simulink model "APF_CTL_VIS_Obs_2023a"  (R2023a)
settings: Solver=ode4  StartTime=0.0  StopTime=tsim  FixedStep=baseRate  RelTol=1e-6  AbsTol=1e-6
values from neighbouring files (symbols this model uses):
  A = [0 0 0 1 0 0 ... (first row only)    [CTL_NEW.m]    (also in UKF_SPOT.m = [1 0 0 dt 0 0)
  a = 25.028    [CTL_NEW.m]
  a1 = shape(1)    [Cardioid.m]    (also in Run_Initializer.m = 0.3)
  a2 = shape(2)    [Cardioid.m]    (also in Run_Initializer.m = 0.3)
  a3 = shape(3)    [Cardioid.m]    (also in Run_Initializer.m = 0.4)
  adadelta_epsilon = 1e-5    (= 1e-05)    [Run_Initializer.m]
  adadelta_gamma = 0.37    [Run_Initializer.m]
  adagrad_epsilon = 1e-8    (= 1e-08)    [Run_Initializer.m]
  adagrad_eta = 0.18    [Run_Initializer.m]
  adam_beta_1 = 0.99    [Run_Initializer.m]
  adam_beta_2 = 0.999    [Run_Initializer.m]
  adam_epsilon = 1e-2    (= 0.01)    [Run_Initializer.m]
  adam_eta = 0.0163    [Run_Initializer.m]
  adamax_beta_1 = 0.5    [Run_Initializer.m]
  adamax_beta_2 = 0.999    [Run_Initializer.m]
  adamax_eta = 0.014    [Run_Initializer.m]
  alpha_Black = 0.9    [UKF_SPOT.m]
  alpha_Blue = 0.9    [UKF_SPOT.m]
  Att_Mode = 0    [Run_Initializer.m]
  b1 = shape(4)    [Cardioid.m]    (also in Run_Initializer.m = 0.175)
  b2 = shape(5)    [Cardioid.m]    (also in Run_Initializer.m = 0.175)
  beta_Black = 2    [UKF_SPOT.m]
  beta_Blue = 20    [UKF_SPOT.m]
  Binv = inv(B)    [Run_Initializer.m]
  BLACK_end = [2, 1.4, deg2rad(368)]    [Run_Initializer.m]
  BLACK_ini = [2, 1.4, deg2rad(188), 0, 0, deg2rad(1.5)]    [Run_Initializer.m]
  BLUE_end = [1.3, 1.25, deg2rad(90)]    [Run_Initializer.m]
  BLUE_ini = [1.3, 1.25, deg2rad(270), 0, 0, deg2rad(-1.5)]    [Run_Initializer.m]
  drop_states_BLACK = BLACK_ini(1:3)    [Run_Initializer.m]
  drop_states_BLUE = BLUE_ini(1:3)    [Run_Initializer.m]
  drop_states_RED = RED_ini(1:3)    [Run_Initializer.m]
  dt = 0.01    [UKF_SPOT.m]
  end_time_black = 300    [Run_Initializer.m]
  end_time_blue = 300    [Run_Initializer.m]
  F_max = 0.22    [CTL_NEW.m]
  Gamma1_el = 0.12    [Run_Initializer.m]
  Gamma1_sh = 0.005    [Run_Initializer.m]
  Gamma1_wr = 0.025    [Run_Initializer.m]
  Gamma2_el = 5    [Run_Initializer.m]
  Gamma2_sh = 5    [Run_Initializer.m]
  Gamma2_wr = 5    [Run_Initializer.m]
  Gamma3_el = 10    [Run_Initializer.m]
  Gamma3_sh = 40    [Run_Initializer.m]
  Gamma3_wr = 40    [Run_Initializer.m]
  Gamma4_el = 0.039    [Run_Initializer.m]
  Gamma4_sh = 0.015    [Run_Initializer.m]
  Gamma4_wr = 0.029    [Run_Initializer.m]
  Gamma5_el = 800    [Run_Initializer.m]
  Gamma5_sh = 800    [Run_Initializer.m]
  Gamma5_wr = 800    [Run_Initializer.m]
  Gamma6_el = 0.000001    (= 1e-06)    [Run_Initializer.m]
  Gamma6_sh = 0.005    [Run_Initializer.m]
  Gamma6_wr = 0.02    [Run_Initializer.m]
  H = [1 0 0 0 0 0 ... (first row only)    [UKF_SPOT.m]
  home_states_BLACK = BLACK_ini(1:3)    [Run_Initializer.m]
  home_states_BLUE = BLUE_ini(1:3)    [Run_Initializer.m]
  home_states_RED = RED_ini(1:3)    [Run_Initializer.m]
  Hz = 0.01    [CTL_NEW.m]
  init_states_BLACK = BLACK_ini(1:3)    [Run_Initializer.m]
  init_states_BLUE = BLUE_ini(1:3)    [Run_Initializer.m]
  init_states_RED = RED_ini(1:3)    [Run_Initializer.m]
  J = IRED    [CTL_NEW.m]    (also in UKF_SPOT.m = 0.20184)
  k = lqr(A,B1,Q,R)    [CTL_NEW.m]
  k_1_0 = k(1,1)    [CTL_NEW.m]
  k_1_t_0 = k(3,3)    [CTL_NEW.m]
  k_2_0 = k(1,4)    [CTL_NEW.m]
  k_2_t_0 = k(3,6)    [CTL_NEW.m]
  K_a = diag([2 2 3.5])    [Run_Initializer.m]
  ka = 1    [Run_Initializer.m]
  Kd_elarm = 0.8    [Run_Initializer.m]
  Kd_sharm = 1.0    (= 1)    [Run_Initializer.m]
  Kd_t = 9.5    [CTL_NEW.m]    (also in Run_Initializer.m)
  Kd_wrarm = 0.6    [Run_Initializer.m]
  Kd_x = 28    [CTL_NEW.m]    (also in Run_Initializer.m)
  Kd_y = Kd_x    (= 28)    [CTL_NEW.m]    (also in Run_Initializer.m)
  Kp_elarm = 1.2    [Run_Initializer.m]
  Kp_sharm = 1.5    [Run_Initializer.m]
  Kp_t = 1    [CTL_NEW.m]    (also in Run_Initializer.m)
  Kp_wrarm = 2    [Run_Initializer.m]
  Kp_x = 3.5    [CTL_NEW.m]    (also in Run_Initializer.m)
  Kp_y = Kp_x    (= 3.5)    [CTL_NEW.m]    (also in Run_Initializer.m)
  kr = 2    [Run_Initializer.m]
  lambda1 = 0.4    [CTL_NEW.m]
  lambda12 = 0.4    [CTL_NEW.m]
  lambda12_t = 0.05    [CTL_NEW.m]
  lambda1_t = 0.05    [CTL_NEW.m]
  lambda2 = 0.4    [CTL_NEW.m]
  lambda2_t = 0.05    [CTL_NEW.m]
  lamda_Black = (alpha_Black^2)*(N + kappa_Black) - N    (= 15.06)    [UKF_SPOT.m]
  lamda_Blue = (alpha_Blue^2)*(N + kappa_Blue) - N    (= 6.96)    [UKF_SPOT.m]
  m = mRED    [CTL_NEW.m]    (also in UKF_SPOT.m = 11.21)
  method = 1    [UKF_SPOT.m]
  Method = 8    [Run_Initializer.m]
  momentum_eta = 0.7    [Run_Initializer.m]
  momentum_gamma = 0.7    [Run_Initializer.m]
  nesterov_eta = 0.6    [Run_Initializer.m]
  nesterov_gamma = 0.3    [Run_Initializer.m]
  Nmat = diag([1 1 1])    [Run_Initializer.m]
  p = 0.4    [CTL_NEW.m]
  P_b = diag([45 45 0])    [Run_Initializer.m]
  P_IC_Black = 0.2*eye(6)    [UKF_SPOT.m]
  P_IC_Blue = 0.2*eye(6)    [UKF_SPOT.m]
  p_t = 0.05    [CTL_NEW.m]
  psi = 1    [Run_Initializer.m]
  PWMFreq = 5    [Run_Initializer.m]
  Q = [w 0 0 0 0 0 ... (first row only)    [CTL_NEW.m]
  Q_a = diag([5, 5, 0])    [Run_Initializer.m]
  Q_b = diag([0.0125, 0.0125, 0.05])    [Run_Initializer.m]
  Q_Black = [0.0000005 0 0 0 0 0 ... (first row only)    [UKF_SPOT.m]
  Q_Blue = [0.000075 0 0 0 0 0 ... (first row only)    [UKF_SPOT.m]
  R = [r 0 0 ... (first row only)    [CTL_NEW.m]
  R_Black = [variance 0 0 ... (first row only)    [UKF_SPOT.m]
  R_Blue = [variance 0 0 ... (first row only)    [UKF_SPOT.m]
  r_hold = 0.427    [Run_Initializer.m]
  r_off = 0.165    [Run_Initializer.m]
  RED_ini = [2.7, 0.4, deg2rad(135+360), 0, 0, 0]    [Run_Initializer.m]
  Red_Rate = 0.025    [CTL_NEW.m]
  RMSprop_epsilon = 1e-8    (= 1e-08)    [Run_Initializer.m]
  RMSprop_eta = 0.025    [Run_Initializer.m]
  RMSprop_gamma = 0.9    [Run_Initializer.m]
  ... (+11 more)
undefined symbols (not defined in the file or in its folder): alpha, alpha_m, alphap, alphat, Am, b, b0, b3, baseRate, beta, Bm, c, Cm, d, DiscIntNeverNeededParam, Dm, drop_states_ARM, epsilon, F_Black_X_nominal, F_Black_Y_nominal, F_Blue_X_nominal, F_Blue_Y_nominal, F_red_X_nominal, F_red_Y_nominal, F_thrusters_BLACK, F_thrusters_BLUE, F_thrusters_RED, IBLACK, IBLUE, IDIST, IEE, IPROX, IRED, K, k1, k1t, k2, k2t, K_t, Kd_tb, Kd_tblue, Kd_tr, Kd_xb, Kd_xblue, Kd_xr, Kd_yb, Kd_yblue, Kd_yr, Kp_tb, Kp_tblue, Kp_tr, Kp_xb, Kp_xblue, Kp_xr, Kp_yb, Kp_yblue, Kp_yr, lamda ... (+34)
libraries: nvidiaSharedBlocks x10, MainLibrary x4, dspsigops x4, simulink x2, etargetslib x1
(part 11 of 15)

== system APF_CTL_VIS_Obs_2023a/Phase #3: Experiment/Change RED Behavior/Sub-Phase #3 /Custom Discrete PD (Attitude)/x_dot -> x2/Hold this value ==
  In1 : Inport
  Action Port : ActionPort  ActionPortLabel=if(u1 ~= 0)
  Out1 : Outport  VectorParamsAs1DForOutWhenUnconnected=off
  wires:
  In1/1 -> Out1/1

== system APF_CTL_VIS_Obs_2023a/Phase #3: Experiment/Change RED Behavior/Sub-Phase #3 /Custom Discrete PD (X-Position)/x_dot -> x2/Hold this value ==
  In1 : Inport
  Action Port : ActionPort  ActionPortLabel=if(u1 ~= 0)
  Out1 : Outport  VectorParamsAs1DForOutWhenUnconnected=off
  wires:
  In1/1 -> Out1/1

== system APF_CTL_VIS_Obs_2023a/Phase #3: Experiment/Change RED Behavior/Sub-Phase #3 /Custom Discrete PD (Y-Position)/x_dot -> x2/Hold this value ==
  In1 : Inport
  Action Port : ActionPort  ActionPortLabel=if(u1 ~= 0)
  Out1 : Outport  VectorParamsAs1DForOutWhenUnconnected=off
  wires:
  In1/1 -> Out1/1

== system APF_CTL_VIS_Obs_2023a/Phase #3: Experiment/Change RED Behavior/Sub-Phase #3 /RED+ARM/Simulated Position Controller/Custom Discrete PD (Elbow) ==
  ey : Inport
  Sum3 : Sum
  kd_elarm : Gain  Gain=Kd_elarm
  kp_elarm : Gain  Gain=Kp_elarm
  "x_dot -> x2" : Subsystem
  Fy : Outport  VectorParamsAs1DForOutWhenUnconnected=off
  wires:
  kd_elarm/1 -> Sum3/1
  Sum3/1 -> Fy/1
  kp_elarm/1 -> Sum3/2
  "x_dot -> x2"/1(dy(t)/dt) -> kd_elarm/1
  ey/1 -> "x_dot -> x2"/1(y(t)), kp_elarm/1

== system APF_CTL_VIS_Obs_2023a/Phase #3: Experiment/Change RED Behavior/Sub-Phase #3 /RED+ARM/Simulated Position Controller/Custom Discrete PD (Shoulder) ==
  ex : Inport
  Sum3 : Sum
  kd_sharm : Gain  Gain=Kd_sharm
  kp_sharm : Gain  Gain=Kp_sharm
  "x_dot -> x2" : Subsystem
  Fx : Outport  VectorParamsAs1DForOutWhenUnconnected=off
  wires:
  kd_sharm/1 -> Sum3/1
  ex/1 -> "x_dot -> x2"/1(y(t)), kp_sharm/1
  kp_sharm/1 -> Sum3/2
  "x_dot -> x2"/1(dy(t)/dt) -> kd_sharm/1
  Sum3/1 -> Fx/1

== system APF_CTL_VIS_Obs_2023a/Phase #3: Experiment/Change RED Behavior/Sub-Phase #3 /RED+ARM/Simulated Position Controller/Custom Discrete PD (Wrist) ==
  ey : Inport
  Sum3 : Sum
  kd_wrarm : Gain  Gain=Kd_wrarm
  kp_wrarm : Gain  Gain=Kp_wrarm
  "x_dot -> x2" : Subsystem
  Fy : Outport  VectorParamsAs1DForOutWhenUnconnected=off
  wires:
  kd_wrarm/1 -> Sum3/1
  Sum3/1 -> Fy/1
  kp_wrarm/1 -> Sum3/2
  "x_dot -> x2"/1(dy(t)/dt) -> kd_wrarm/1
  ey/1 -> "x_dot -> x2"/1(y(t)), kp_wrarm/1

== system APF_CTL_VIS_Obs_2023a/Phase #3: Experiment/Change RED Behavior/Sub-Phase #4/CTL/If Action Subsystem/CSMC3 ==
  note: epsilon = 2*u_max
  note: k = mass, but i may make it variable for performance
  note: alpha = variable
  e_x : Inport
  e_y : Inport  Port=2
  e_t : Inport  Port=3
  Derivative : Derivative
  Derivative1 : Derivative
  Derivative2 : Derivative
  MATLAB Function : MATLAB Function  TreatAsAtomicUnit=on
  MATLAB Function1 : MATLAB Function  TreatAsAtomicUnit=on
  MATLAB Function2 : MATLAB Function  TreatAsAtomicUnit=on
  MATLAB Function3 : MATLAB Function  TreatAsAtomicUnit=on
  MATLAB Function4 : MATLAB Function  TreatAsAtomicUnit=on
  MATLAB Function5 : MATLAB Function  TreatAsAtomicUnit=on
  MATLAB Function6 : MATLAB Function  TreatAsAtomicUnit=on
  MATLAB Function7 : MATLAB Function  TreatAsAtomicUnit=on
  MATLAB Function8 : MATLAB Function  TreatAsAtomicUnit=on
  Saturation{,1..5} (6 alike) : Saturate  UpperLimit=epsilon  LowerLimit=-epsilon
  Sum : Sum  Inputs=++|
  Sum1 : Sum  Inputs=++|
  Sum2 : Sum  Inputs=++|
  F_x : Outport
  F_y : Outport  Port=2
  tau : Outport  Port=3
  wires:
  Sum2/1 -> tau/1
  MATLAB Function6/1(u) -> Saturation5/1
  MATLAB Function8/1(phi) -> MATLAB Function6/1(phi)
  Derivative2/1 -> MATLAB Function8/2(q2), MATLAB Function7/1(q2)
  Saturation5/1 -> Sum2/1
  Saturation4/1 -> Sum2/2
  MATLAB Function7/1(u) -> Saturation4/1
  e_t/1 -> Derivative2/1, MATLAB Function8/1(q1)
  Sum1/1 -> F_y/1
  MATLAB Function3/1(u) -> Saturation3/1
  MATLAB Function4/1(u) -> Saturation2/1
  Derivative1/1 -> MATLAB Function4/1(q2), MATLAB Function5/2(q2)
  e_y/1 -> MATLAB Function5/1(q1), Derivative1/1
  Saturation3/1 -> Sum1/1
  MATLAB Function5/1(phi) -> MATLAB Function3/1(phi)
  Saturation2/1 -> Sum1/2
  Saturation1/1 -> Sum/1
  Saturation/1 -> Sum/2
  MATLAB Function2/1(phi) -> MATLAB Function/1(phi)
  MATLAB Function1/1(u) -> Saturation/1
  MATLAB Function/1(u) -> Saturation1/1
  Sum/1 -> F_x/1
  Derivative/1 -> MATLAB Function1/1(q2), MATLAB Function2/2(q2)
  e_x/1 -> Derivative/1, MATLAB Function2/1(q1)

== system APF_CTL_VIS_Obs_2023a/Phase #3: Experiment/Change RED Behavior/Sub-Phase #4/CTL/If Action Subsystem/DAC Controller1 ==
  e_x : Inport
  In2 : Inport  Port=2
  e_t : Inport  Port=3
  Add2 : Sum
  Derivative1 : Derivative
  Derivative2 : Derivative
  Derivative3 : Derivative
  Discrete-Time Integrator : DiscreteIntegrator  InitialCondition=k_2_t_0  SampleTime=-1  ICPrevOutput=DiscIntNeverNeededParam  ICPrevScaledInput=DiscIntNeverNeededParam
  Discrete-Time Integrator1 : DiscreteIntegrator  InitialCondition=k_1_t_0  SampleTime=-1  ICPrevOutput=DiscIntNeverNeededParam  ICPrevScaledInput=DiscIntNeverNeededParam
  Discrete-Time Integrator2 : DiscreteIntegrator  InitialCondition=k_2_0  SampleTime=-1  ICPrevOutput=DiscIntNeverNeededParam  ICPrevScaledInput=DiscIntNeverNeededParam
  Discrete-Time Integrator3 : DiscreteIntegrator  InitialCondition=k_1_0  SampleTime=-1  ICPrevOutput=DiscIntNeverNeededParam  ICPrevScaledInput=DiscIntNeverNeededParam
  Discrete-Time Integrator4 : DiscreteIntegrator  InitialCondition=k_2_0  SampleTime=-1  ICPrevOutput=DiscIntNeverNeededParam  ICPrevScaledInput=DiscIntNeverNeededParam
  Discrete-Time Integrator5 : DiscreteIntegrator  InitialCondition=k_1_0  SampleTime=-1  ICPrevOutput=DiscIntNeverNeededParam  ICPrevScaledInput=DiscIntNeverNeededParam
  Fx Gain Derivatives : MATLAB Function  TreatAsAtomicUnit=on
  Fy Gain Derivatives : MATLAB Function  TreatAsAtomicUnit=on
  Product4 : Product
  Product5 : Product
  Pseudo Derivative2 : TransferFcn  Commented=on  Numerator=[a 0]  Denominator=[1 a]
  Torque Gain Derivatives : MATLAB Function  TreatAsAtomicUnit=on
  k_1*q_1_x : Product
  k_1*q_1_y : Product
  k_2*q2_x : Product
  k_2*q2_y : Product
  u_x : Sum
  u_y : Sum
  Out1 : Outport
  Out2 : Outport  Port=2
  Out3 : Outport  Port=3
  wires:
  u_y/1 -> Out2/1
  Discrete-Time Integrator3/1 -> k_1*q_1_y/1
  Derivative1/1 -> k_2*q2_y/1, Fy Gain Derivatives/1(e_ydot)
  In2/1 -> Derivative1/1, Fy Gain Derivatives/2(e_y), k_1*q_1_y/2
  k_2*q2_y/1 -> u_y/1
  Fy Gain Derivatives/2(k1_dot) -> Discrete-Time Integrator3/1
  Discrete-Time Integrator2/1 -> k_2*q2_y/2
  k_1*q_1_y/1 -> u_y/2
  Fy Gain Derivatives/1(k2_dot) -> Discrete-Time Integrator2/1
  Discrete-Time Integrator1/1 -> Product5/2
  Torque Gain Derivatives/1(k1_dot) -> Discrete-Time Integrator1/1
  Derivative3/1 -> Product4/2, Torque Gain Derivatives/2(e_tdot)
  Discrete-Time Integrator/1 -> Product4/1
  Product5/1 -> Add2/1
  Product4/1 -> Add2/2
  Torque Gain Derivatives/2(k2_dot) -> Discrete-Time Integrator/1
  Add2/1 -> Out3/1
  e_x/1 -> Derivative2/1, k_1*q_1_x/2, Fx Gain Derivatives/2(e_x)
  Discrete-Time Integrator4/1 -> k_2*q2_x/2
  Discrete-Time Integrator5/1 -> k_1*q_1_x/1
  Fx Gain Derivatives/2(k1_dot) -> Discrete-Time Integrator5/1
  Fx Gain Derivatives/1(k2_dot) -> Discrete-Time Integrator4/1
  Derivative2/1 -> k_2*q2_x/1, Fx Gain Derivatives/1(e_xdot)
  k_1*q_1_x/1 -> u_x/2
  u_x/1 -> Out1/1
  k_2*q2_x/1 -> u_x/1
  e_t/1 -> Product5/1, Derivative3/1, Torque Gain Derivatives/1(e_t)

== system APF_CTL_VIS_Obs_2023a/Phase #3: Experiment/Change RED Behavior/Sub-Phase #4/CTL/If Action Subsystem/DAC Controller2 ==
  e_x : Inport
  In2 : Inport  Port=2
  e_t : Inport  Port=3
  Add2 : Sum
  Derivative1 : Derivative
  Derivative2 : Derivative
  Derivative3 : Derivative
  Discrete-Time Integrator : DiscreteIntegrator  InitialCondition=k_2_t_0  SampleTime=-1  ICPrevOutput=DiscIntNeverNeededParam  ICPrevScaledInput=DiscIntNeverNeededParam
  Discrete-Time Integrator1 : DiscreteIntegrator  InitialCondition=k_1_t_0  SampleTime=-1  ICPrevOutput=DiscIntNeverNeededParam  ICPrevScaledInput=DiscIntNeverNeededParam
  Discrete-Time Integrator2 : DiscreteIntegrator  InitialCondition=k_2_0  SampleTime=-1  ICPrevOutput=DiscIntNeverNeededParam  ICPrevScaledInput=DiscIntNeverNeededParam
  Discrete-Time Integrator3 : DiscreteIntegrator  InitialCondition=k_1_0  SampleTime=-1  ICPrevOutput=DiscIntNeverNeededParam  ICPrevScaledInput=DiscIntNeverNeededParam
  Discrete-Time Integrator4 : DiscreteIntegrator  InitialCondition=k_2_0  SampleTime=-1  ICPrevOutput=DiscIntNeverNeededParam  ICPrevScaledInput=DiscIntNeverNeededParam
  Discrete-Time Integrator5 : DiscreteIntegrator  InitialCondition=k_1_0  SampleTime=-1  ICPrevOutput=DiscIntNeverNeededParam  ICPrevScaledInput=DiscIntNeverNeededParam
  Fx Gain Derivatives : MATLAB Function  TreatAsAtomicUnit=on
  Fy Gain Derivatives : MATLAB Function  TreatAsAtomicUnit=on
  Product4 : Product
  Product5 : Product
  Pseudo Derivative2 : TransferFcn  Commented=on  Numerator=[a 0]  Denominator=[1 a]
  Torque Gain Derivatives : MATLAB Function  TreatAsAtomicUnit=on
  k_1*q_1_x : Product
  k_1*q_1_y : Product
  k_2*q2_x : Product
  k_2*q2_y : Product
  u_x : Sum
  u_y : Sum
  Out1 : Outport
  Out2 : Outport  Port=2
  Out3 : Outport  Port=3
  wires:
  e_t/1 -> Torque Gain Derivatives/1(e_t), Derivative3/1, Product5/1
  k_2*q2_x/1 -> u_x/1
  u_x/1 -> Out1/1
  k_1*q_1_x/1 -> u_x/2
  Derivative2/1 -> Fx Gain Derivatives/1(e_xdot), k_2*q2_x/1
  Fx Gain Derivatives/1(k2_dot) -> Discrete-Time Integrator4/1
  Fx Gain Derivatives/2(k1_dot) -> Discrete-Time Integrator5/1
  Discrete-Time Integrator5/1 -> k_1*q_1_x/1
  Discrete-Time Integrator4/1 -> k_2*q2_x/2
  e_x/1 -> Fx Gain Derivatives/2(e_x), k_1*q_1_x/2, Derivative2/1
  Add2/1 -> Out3/1
  Torque Gain Derivatives/2(k2_dot) -> Discrete-Time Integrator/1
  Product4/1 -> Add2/2
  Product5/1 -> Add2/1
  Discrete-Time Integrator/1 -> Product4/1
  Derivative3/1 -> Torque Gain Derivatives/2(e_tdot), Product4/2
  Torque Gain Derivatives/1(k1_dot) -> Discrete-Time Integrator1/1
  Discrete-Time Integrator1/1 -> Product5/2
  Fy Gain Derivatives/1(k2_dot) -> Discrete-Time Integrator2/1
  k_1*q_1_y/1 -> u_y/2
  Discrete-Time Integrator2/1 -> k_2*q2_y/2
  Fy Gain Derivatives/2(k1_dot) -> Discrete-Time Integrator3/1
  k_2*q2_y/1 -> u_y/1
  In2/1 -> k_1*q_1_y/2, Fy Gain Derivatives/2(e_y), Derivative1/1
  Derivative1/1 -> Fy Gain Derivatives/1(e_ydot), k_2*q2_y/1
  Discrete-Time Integrator3/1 -> k_1*q_1_y/1
  u_y/1 -> Out2/1

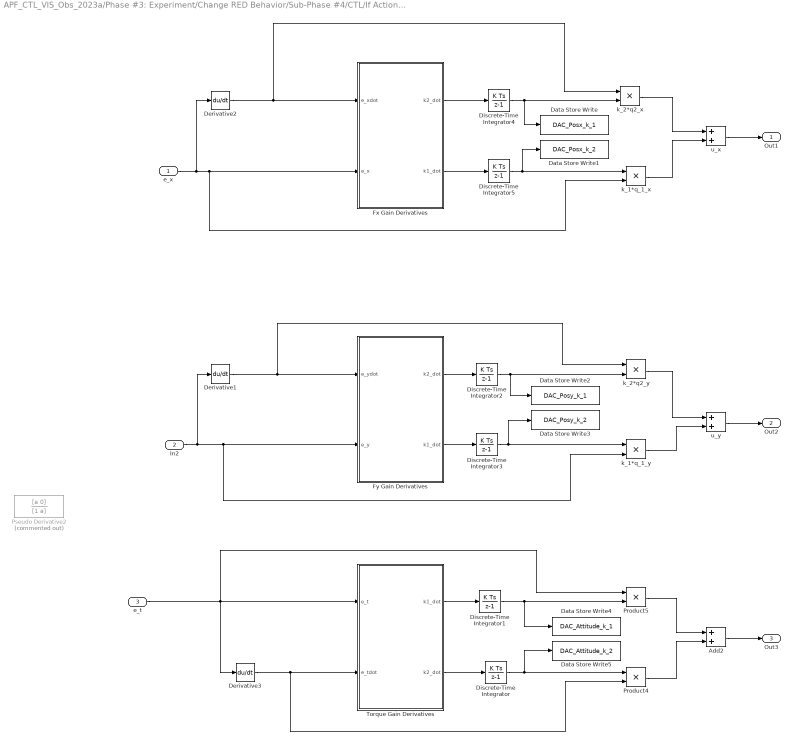
== system APF_CTL_VIS_Obs_2023a/Phase #3: Experiment/Change RED Behavior/Sub-Phase #4/CTL/If Action Subsystem/DAC Controller3 ==
  e_x : Inport
  In2 : Inport  Port=2
  e_t : Inport  Port=3
  Add2 : Sum
  Data Store Write : DataStoreWrite  DataStoreName=DAC_Posx_k_1  IndexOptions=Index vector (dialog)  Indices=1  OutputSizes=1
  Data Store Write1 : DataStoreWrite  DataStoreName=DAC_Posx_k_2  IndexOptions=Index vector (dialog)  Indices=1  OutputSizes=1
  Data Store Write2 : DataStoreWrite  DataStoreName=DAC_Posy_k_1  IndexOptions=Index vector (dialog)  Indices=1  OutputSizes=1
  Data Store Write3 : DataStoreWrite  DataStoreName=DAC_Posy_k_2  IndexOptions=Index vector (dialog)  Indices=1  OutputSizes=1
  Data Store Write4 : DataStoreWrite  DataStoreName=DAC_Attitude_k_1  IndexOptions=Index vector (dialog)  Indices=1  OutputSizes=1
  Data Store Write5 : DataStoreWrite  DataStoreName=DAC_Attitude_k_2  IndexOptions=Index vector (dialog)  Indices=1  OutputSizes=1
  Derivative1 : Derivative
  Derivative2 : Derivative
  Derivative3 : Derivative
  Discrete-Time Integrator : DiscreteIntegrator  InitialCondition=k_2_t_0  SampleTime=-1  ICPrevOutput=DiscIntNeverNeededParam  ICPrevScaledInput=DiscIntNeverNeededParam
  Discrete-Time Integrator1 : DiscreteIntegrator  InitialCondition=k_1_t_0  SampleTime=-1  ICPrevOutput=DiscIntNeverNeededParam  ICPrevScaledInput=DiscIntNeverNeededParam
  Discrete-Time Integrator2 : DiscreteIntegrator  InitialCondition=k_2_0  SampleTime=-1  ICPrevOutput=DiscIntNeverNeededParam  ICPrevScaledInput=DiscIntNeverNeededParam
  Discrete-Time Integrator3 : DiscreteIntegrator  InitialCondition=k_1_0  SampleTime=-1  ICPrevOutput=DiscIntNeverNeededParam  ICPrevScaledInput=DiscIntNeverNeededParam
  Discrete-Time Integrator4 : DiscreteIntegrator  InitialCondition=k_2_0  SampleTime=-1  ICPrevOutput=DiscIntNeverNeededParam  ICPrevScaledInput=DiscIntNeverNeededParam
  Discrete-Time Integrator5 : DiscreteIntegrator  InitialCondition=k_1_0  SampleTime=-1  ICPrevOutput=DiscIntNeverNeededParam  ICPrevScaledInput=DiscIntNeverNeededParam
  Fx Gain Derivatives : MATLAB Function  TreatAsAtomicUnit=on
  Fy Gain Derivatives : MATLAB Function  TreatAsAtomicUnit=on
  Product4 : Product
  Product5 : Product
  Pseudo Derivative2 : TransferFcn  Commented=on  Numerator=[a 0]  Denominator=[1 a]
  Torque Gain Derivatives : MATLAB Function  TreatAsAtomicUnit=on
  k_1*q_1_x : Product
  k_1*q_1_y : Product
  k_2*q2_x : Product
  k_2*q2_y : Product
  u_x : Sum
  u_y : Sum
  Out1 : Outport
  Out2 : Outport  Port=2
  Out3 : Outport  Port=3
  wires:
  u_y/1 -> Out2/1
  Discrete-Time Integrator3/1 -> Data Store Write3/1, k_1*q_1_y/1
  Derivative1/1 -> k_2*q2_y/1, Fy Gain Derivatives/1(e_ydot)
  In2/1 -> Derivative1/1, Fy Gain Derivatives/2(e_y), k_1*q_1_y/2
  k_2*q2_y/1 -> u_y/1
  Fy Gain Derivatives/2(k1_dot) -> Discrete-Time Integrator3/1
  Discrete-Time Integrator2/1 -> Data Store Write2/1, k_2*q2_y/2
  k_1*q_1_y/1 -> u_y/2
  Fy Gain Derivatives/1(k2_dot) -> Discrete-Time Integrator2/1
  Discrete-Time Integrator1/1 -> Data Store Write4/1, Product5/2
  Torque Gain Derivatives/1(k1_dot) -> Discrete-Time Integrator1/1
  Derivative3/1 -> Product4/2, Torque Gain Derivatives/2(e_tdot)
  Discrete-Time Integrator/1 -> Data Store Write5/1, Product4/1
  Product5/1 -> Add2/1
  Product4/1 -> Add2/2
  Torque Gain Derivatives/2(k2_dot) -> Discrete-Time Integrator/1
  Add2/1 -> Out3/1
  e_x/1 -> Derivative2/1, k_1*q_1_x/2, Fx Gain Derivatives/2(e_x)
  Discrete-Time Integrator4/1 -> Data Store Write/1, k_2*q2_x/2
  Discrete-Time Integrator5/1 -> Data Store Write1/1, k_1*q_1_x/1
  Fx Gain Derivatives/2(k1_dot) -> Discrete-Time Integrator5/1
  Fx Gain Derivatives/1(k2_dot) -> Discrete-Time Integrator4/1
  Derivative2/1 -> k_2*q2_x/1, Fx Gain Derivatives/1(e_xdot)
  k_1*q_1_x/1 -> u_x/2
  u_x/1 -> Out1/1
  k_2*q2_x/1 -> u_x/1
  e_t/1 -> Product5/1, Derivative3/1, Torque Gain Derivatives/1(e_t)

== system APF_CTL_VIS_Obs_2023a/Phase #3: Experiment/Change RED Behavior/Sub-Phase #4/CTL/If Action Subsystem/H_inf ==
  e_x : Inport
  e_y : Inport  Port=2
  e_t : Inport  Port=3
  H Infinity (Attitude) : Subsystem
  H Infinity (X-Position) : Subsystem
  H Infinity (Y-Position) : Subsystem
  F_x : Outport
  F_y : Outport  Port=2
  tau : Outport  Port=3
  wires:
  e_x/1 -> H Infinity (X-Position)/1(ex)
  e_y/1 -> H Infinity (Y-Position)/1(ey)
  e_t/1 -> H Infinity (Attitude)/1(ez)
  H Infinity (Attitude)/1(Tz) -> tau/1
  H Infinity (Y-Position)/1(Fy) -> F_y/1
  H Infinity (X-Position)/1(Fx) -> F_x/1

== system APF_CTL_VIS_Obs_2023a/Phase #3: Experiment/Change RED Behavior/Sub-Phase #4/CTL/If Action Subsystem/Homo ==
  e_x : Inport
  e_y : Inport  Port=2
  e_t : Inport  Port=3
  Derivative : Derivative
  Derivative1 : Derivative
  Derivative2 : Derivative
  MATLAB Function : MATLAB Function  TreatAsAtomicUnit=on
  MATLAB Function1 : MATLAB Function  TreatAsAtomicUnit=on
  MATLAB Function2 : MATLAB Function  TreatAsAtomicUnit=on
  MATLAB Function3 : MATLAB Function  TreatAsAtomicUnit=on
  MATLAB Function4 : MATLAB Function  TreatAsAtomicUnit=on
  MATLAB Function5 : MATLAB Function  TreatAsAtomicUnit=on
  Sum : Sum  Inputs=++|
  Sum1 : Sum  Inputs=++|
  Sum2 : Sum  Inputs=++|
  F_x : Outport
  F_y : Outport  Port=2
  tau : Outport  Port=3
  wires:
  e_x/1 -> Derivative2/1, MATLAB Function/1(q1)
  Derivative2/1 -> MATLAB Function1/1(q2)
  Sum/1 -> F_x/1
  MATLAB Function/1(u) -> Sum/1
  MATLAB Function1/1(u) -> Sum/2
  Derivative1/1 -> MATLAB Function3/1(q2)
  Sum1/1 -> F_y/1
  MATLAB Function3/1(u) -> Sum1/2
  e_y/1 -> Derivative1/1, MATLAB Function2/1(q1)
  MATLAB Function2/1(u) -> Sum1/1
  e_t/1 -> Derivative/1, MATLAB Function4/1(q1)
  Derivative/1 -> MATLAB Function5/1(q2)
  MATLAB Function5/1(u) -> Sum2/2
  MATLAB Function4/1(u) -> Sum2/1
  Sum2/1 -> tau/1

== system APF_CTL_VIS_Obs_2023a/Phase #3: Experiment/Change RED Behavior/Sub-Phase #4/CTL/If Action Subsystem/LQR ==
  e_x : Inport
  e_y : Inport  Port=2
  e_t : Inport  Port=3
  Constant : Constant  Value=k
  Demux : Demux  Outputs=3
  Derivative : Derivative
  Derivative1 : Derivative
  Derivative2 : Derivative
  MATLAB Function : MATLAB Function  TreatAsAtomicUnit=on
  F_x : Outport
  F_y : Outport  Port=2
  tau : Outport  Port=3
  wires:
  Constant/1 -> MATLAB Function/1(k)
  MATLAB Function/1(u) -> Demux/1
  Demux/2 -> F_y/1
  Demux/1 -> F_x/1
  Demux/3 -> tau/1
  e_t/1 -> MATLAB Function/6(q1_t), Derivative/1
  e_y/1 -> Derivative1/1, MATLAB Function/4(q1_y)
  e_x/1 -> Derivative2/1, MATLAB Function/2(q1_x)
  Derivative/1 -> MATLAB Function/7(q2_t)
  Derivative1/1 -> MATLAB Function/5(q2_y)
  Derivative2/1 -> MATLAB Function/3(q2_x)

== system APF_CTL_VIS_Obs_2023a/Phase #3: Experiment/Change RED Behavior/Sub-Phase #4/CTL/If Action Subsystem/PD Controller1 ==
  In1 : Inport
  In2 : Inport  Port=2
  Err : Inport  Port=3
  Derivative : Derivative
  Derivative1 : Derivative
  Derivative2 : Derivative
  Gain : Gain  Gain=Kp_x
  Gain1 : Gain  Gain=Kp_y
  Gain2 : Gain  Gain=Kp_t
  Gain3 : Gain  Gain=Kd_x
  Gain4 : Gain  Gain=Kd_y
  Gain5 : Gain  Gain=Kd_t
  Sum : Sum  Inputs=|++
  Sum1 : Sum  Inputs=|++
  Sum2 : Sum  Inputs=|++
  Out1 : Outport
  Out2 : Outport  Port=2
  Out3 : Outport  Port=3
  wires:
  In1/1 -> Gain3/1, Gain/1
  In2/1 -> Gain4/1, Gain1/1
  Err/1 -> Gain2/1, Gain5/1
  Gain3/1 -> Derivative/1
  Gain4/1 -> Derivative1/1
  Gain5/1 -> Derivative2/1
  Gain/1 -> Sum/1
  Derivative/1 -> Sum/2
  Sum/1 -> Out1/1
  Gain1/1 -> Sum1/1
  Sum1/1 -> Out2/1
  Derivative1/1 -> Sum1/2
  Sum2/1 -> Out3/1
  Gain2/1 -> Sum2/1
  Derivative2/1 -> Sum2/2

== system APF_CTL_VIS_Obs_2023a/Phase #3: Experiment/Change RED Behavior/Sub-Phase #4/CTL/If Action Subsystem/Sat ==
  e_x : Inport
  e_y : Inport  Port=2
  e_t : Inport  Port=3
  Derivative : Derivative
  Derivative1 : Derivative
  Derivative2 : Derivative
  MATLAB Function : MATLAB Function  TreatAsAtomicUnit=on
  MATLAB Function1 : MATLAB Function  TreatAsAtomicUnit=on
  MATLAB Function2 : MATLAB Function  TreatAsAtomicUnit=on
  MATLAB Function3 : MATLAB Function  TreatAsAtomicUnit=on
  MATLAB Function4 : MATLAB Function  TreatAsAtomicUnit=on
  MATLAB Function5 : MATLAB Function  TreatAsAtomicUnit=on
  F_x : Outport
  F_y : Outport  Port=2
  tau : Outport  Port=3
  wires:
  e_x/1 -> Derivative/1, MATLAB Function/2(q1)
  e_y/1 -> MATLAB Function1/2(q1), Derivative1/1
  Derivative1/1 -> MATLAB Function1/1(q2), MATLAB Function4/1(q2)
  e_t/1 -> Derivative2/1, MATLAB Function2/2(q1)
  Derivative2/1 -> MATLAB Function5/1(q2), MATLAB Function2/1(q2)
  Derivative/1 -> MATLAB Function3/1(q2), MATLAB Function/1(q2)
  MATLAB Function/1(saturation) -> MATLAB Function3/2(u)
  MATLAB Function2/1(saturation) -> MATLAB Function5/2(u)
  MATLAB Function1/1(saturation) -> MATLAB Function4/2(u)
  MATLAB Function3/1(saturation) -> F_x/1
  MATLAB Function4/1(saturation) -> F_y/1
  MATLAB Function5/1(saturation) -> tau/1

== system APF_CTL_VIS_Obs_2023a/Phase #3: Experiment/Change RED Behavior/Sub-Phase #4/CTL/Subsystem1/Custom Discrete PD (Attitude) ==
  ez : Inport
  Sum3 : Sum
  kd_tr : Gain  Gain=Kd_tr
  kp_tr : Gain  Gain=Kp_tr
  "x_dot -> x2" : Subsystem
  Tz : Outport  VectorParamsAs1DForOutWhenUnconnected=off
  wires:
  kd_tr/1 -> Sum3/1
  Sum3/1 -> Tz/1
  kp_tr/1 -> Sum3/2
  "x_dot -> x2"/1(dy(t)/dt) -> kd_tr/1
  ez/1 -> "x_dot -> x2"/1(y(t)), kp_tr/1

== system APF_CTL_VIS_Obs_2023a/Phase #3: Experiment/Change RED Behavior/Sub-Phase #4/CTL/Subsystem1/SAT_Angle1 ==
  In1 : Inport
  Add2 : Sum  Commented=on
  Derivative2 : Derivative
  Derivative3 : Derivative  Commented=on
  Discrete-Time Integrator : DiscreteIntegrator  Commented=on  InitialCondition=k_2_t_0  SampleTime=-1  ICPrevOutput=DiscIntNeverNeededParam  ICPrevScaledInput=DiscIntNeverNeededParam
  Discrete-Time Integrator1 : DiscreteIntegrator  Commented=on  InitialCondition=k_1_t_0  SampleTime=-1  ICPrevOutput=DiscIntNeverNeededParam  ICPrevScaledInput=DiscIntNeverNeededParam
  MATLAB Function2 : MATLAB Function  TreatAsAtomicUnit=on
  MATLAB Function5 : MATLAB Function  TreatAsAtomicUnit=on
  Product4 : Product  Commented=on
  Product5 : Product  Commented=on
  Torque Gain Derivatives : MATLAB Function  Commented=on  TreatAsAtomicUnit=on
  Out1 : Outport
  wires:
  MATLAB Function5/1(saturation) -> Out1/1
  In1/1 -> Derivative2/1, MATLAB Function2/2(q1)
  Product4/1 -> Add2/2
  Torque Gain Derivatives/1(k1_dot) -> Discrete-Time Integrator1/1
  Discrete-Time Integrator1/1 -> Product5/2
  Product5/1 -> Add2/1
  Torque Gain Derivatives/2(k2_dot) -> Discrete-Time Integrator/1
  Derivative3/1 -> Torque Gain Derivatives/2(e_tdot), Product4/2
  Discrete-Time Integrator/1 -> Product4/1
  MATLAB Function2/1(saturation) -> MATLAB Function5/2(u)
  Derivative2/1 -> MATLAB Function2/1(q2), MATLAB Function5/1(q2)

== system APF_CTL_VIS_Obs_2023a/Phase #3: Experiment/Change RED Behavior/Sub-Phase #4/CTL/Subsystem1/Subsystem ==
  um : Inport
  state_red : Inport  Port=2
  Demux : Demux  Outputs=2
  Demux1 : Demux
  Demux2 : Demux  Commented=on  Outputs=2
  Derivative : Derivative  Commented=on
  Derivative1 : Derivative  Commented=on
  Ideal Plant Model1 : Subsystem
  Mux1 : Mux  Commented=on
  Plant Output : Subsystem
  RED_um1 : DataStoreWrite  DataStoreName=um_x  IndexOptions=Index vector (dialog)  Indices=1  OutputSizes=1
  RED_um2 : DataStoreWrite  Commented=on  DataStoreName=um_y  IndexOptions=Index vector (dialog)  Indices=1  OutputSizes=1
  RED_xm : DataStoreWrite  DataStoreName=xm_1  IndexOptions=Index vector (dialog)  Indices=1  OutputSizes=1
  RED_xm1 : DataStoreWrite  Commented=on  DataStoreName=xm_2  IndexOptions=Index vector (dialog)  Indices=1  OutputSizes=1
  RED_xm2 : DataStoreWrite  Commented=on  DataStoreName=xm_3  IndexOptions=Index vector (dialog)  Indices=1  OutputSizes=1
  RED_xm3 : DataStoreWrite  Commented=on  DataStoreName=xm_4  IndexOptions=Index vector (dialog)  Indices=1  OutputSizes=1
  SAC Ctl : Subsystem
  Sum1 : Sum  Inputs=|+-
  u : Outport
  wires:
  Sum1/1 -> SAC Ctl/3(ey)
  state_red/1 -> Plant Output/1(In1)
  SAC Ctl/1(u) -> u/1
  Plant Output/1(Out1) -> Sum1/2
  Ideal Plant Model1/1(ym) -> Sum1/1
  Demux/1 -> RED_um1/1
  Demux/2 -> RED_um2/1
  Demux1/1 -> RED_xm/1
  Demux1/2 -> RED_xm1/1
  Demux1/3 -> RED_xm2/1
  Demux1/4 -> RED_xm3/1
  um/1 -> Demux/1, Ideal Plant Model1/1(um), SAC Ctl/1(um)
  Demux2/1 -> Derivative/1, Mux1/1
  Demux2/2 -> Derivative1/1, Mux1/2
  Derivative1/1 -> Mux1/4
  Derivative/1 -> Mux1/3
  Ideal Plant Model1/2(xm) -> Demux1/1, SAC Ctl/2(xm)

== system APF_CTL_VIS_Obs_2023a/Phase #3: Experiment/Change RED Behavior/Sub-Phase #4/CTL/Target Finder/LQR1 ==
  e_x : Inport
  e_y : Inport  Port=2
  e_t : Inport  Port=3
  Constant : Constant  Value=k
  Demux : Demux  Outputs=3
  MATLAB Function : MATLAB Function  TreatAsAtomicUnit=on
  Pseudo Derivative : TransferFcn  Numerator=[a 0]  Denominator=[1 a]
  Pseudo Derivative1 : TransferFcn  Numerator=[a 0]  Denominator=[1 a]
  Pseudo Derivative2 : TransferFcn  Numerator=[a 0]  Denominator=[1 a]
  F_x : Outport
  F_y : Outport  Port=2
  tau : Outport  Port=3
  wires:
  Pseudo Derivative/1 -> MATLAB Function/3(q2_x)
  Pseudo Derivative1/1 -> MATLAB Function/5(q2_y)
  Pseudo Derivative2/1 -> MATLAB Function/7(q2_t)
  e_x/1 -> MATLAB Function/2(q1_x), Pseudo Derivative/1
  e_y/1 -> MATLAB Function/4(q1_y), Pseudo Derivative1/1
  e_t/1 -> MATLAB Function/6(q1_t), Pseudo Derivative2/1
  Demux/3 -> tau/1
  Demux/1 -> F_x/1
  Demux/2 -> F_y/1
  MATLAB Function/1(u) -> Demux/1
  Constant/1 -> MATLAB Function/1(k)

== system APF_CTL_VIS_Obs_2023a/Phase #3: Experiment/Change RED Behavior/Sub-Phase #4/CTL/Target Tracker/LQR1 ==
  e_x : Inport
  e_y : Inport  Port=2
  e_t : Inport  Port=3
  Constant : Constant  Value=k
  Demux : Demux  Outputs=3
  MATLAB Function : MATLAB Function  TreatAsAtomicUnit=on
  Pseudo Derivative : TransferFcn  Numerator=[a 0]  Denominator=[1 a]
  Pseudo Derivative1 : TransferFcn  Numerator=[a 0]  Denominator=[1 a]
  Pseudo Derivative2 : TransferFcn  Numerator=[a 0]  Denominator=[1 a]
  F_x : Outport
  F_y : Outport  Port=2
  tau : Outport  Port=3
  wires:
  Pseudo Derivative/1 -> MATLAB Function/3(q2_x)
  Pseudo Derivative1/1 -> MATLAB Function/5(q2_y)
  Pseudo Derivative2/1 -> MATLAB Function/7(q2_t)
  e_x/1 -> MATLAB Function/2(q1_x), Pseudo Derivative/1
  e_y/1 -> MATLAB Function/4(q1_y), Pseudo Derivative1/1
  e_t/1 -> MATLAB Function/6(q1_t), Pseudo Derivative2/1
  Demux/3 -> tau/1
  Demux/1 -> F_x/1
  Demux/2 -> F_y/1
  MATLAB Function/1(u) -> Demux/1
  Constant/1 -> MATLAB Function/1(k)

== system APF_CTL_VIS_Obs_2023a/Phase #3: Experiment/Change RED Behavior/Sub-Phase #4/GDC/APF/GDC ==
  IsBlue : Inport
  state_red : Inport  Port=2
  state_black : Inport  Port=3
  state_blue : Inport  Port=4
  MATLAB Function : MATLAB Function  TreatAsAtomicUnit=on
  Reshape : Reshape
  Reshape1 : Reshape
  Subsystem1 : Subsystem
  To Workspace : ToWorkspace  VariableName=desired  SampleTime=-1
  To Workspace1 : ToWorkspace  VariableName=phi_tot  SampleTime=-1
  To Workspace2 : ToWorkspace  VariableName=desired_path  SampleTime=-1
  To Workspace3 : ToWorkspace  VariableName=state_red_control_n  SampleTime=-1
  To Workspace4 : ToWorkspace  VariableName=phi_tot_grad  SampleTime=-1
  path : Outport
  u : Outport  Port=2
  wires:
  MATLAB Function/2(phi_tot_grad) -> To Workspace4/1, Subsystem1/2(phi_tot_grad)
  Reshape/1 -> To Workspace3/1
  MATLAB Function/3(u) -> u/1
  state_black/1 -> Subsystem1/3(state_black), MATLAB Function/2(state_black)
  state_red/1 -> Subsystem1/1(state_red), MATLAB Function/1(state_red), Reshape/1
  state_blue/1 -> Subsystem1/4(state_blue), MATLAB Function/3(state_blue)
  MATLAB Function/1(phi_tot) -> To Workspace1/1
  Subsystem1/1(Path) -> Reshape1/1, path/1
  MATLAB Function/4(state_desired) -> To Workspace/1
  Reshape1/1 -> To Workspace2/1
  IsBlue/1 -> Subsystem1/5(isBlue), MATLAB Function/4(IsBlue)

== system APF_CTL_VIS_Obs_2023a/Phase #3: Experiment/Change RED Behavior/Sub-Phase #4/GDC/Target Finder/Constant Angular Rate ==
  Constant : Constant  Value=RED_ini(3)
  Desired Rate (RED) : Constant  Value=Red_Rate  SampleTime=-1
  Gain : Gain  Gain=-1
  Product : Product
  Subsystem : Subsystem
  Sum : Sum  Inputs=|++
  Wrap1 : Subsystem
  Out1 : Outport
  wires:
  Constant/1 -> Sum/2
  Wrap1/1(wrapped) -> Sum/1
  Desired Rate (RED)/1 -> Gain/1
  Subsystem/1(Time) -> Product/2
  Sum/1 -> Out1/1
  Product/1 -> Wrap1/1(unwrapped)
  Gain/1 -> Product/1

== system APF_CTL_VIS_Obs_2023a/Phase #3: Experiment/Change RED Behavior/Sub-Phase #4/GDC/Target Finder/Hold Position ==
  Constant1 : Constant  Value=RED_ini(1)
  Constant2 : Constant  Value=RED_ini(2)
  Out1 : Outport
  Out2 : Outport  Port=2
  wires:
  Constant1/1 -> Out1/1
  Constant2/1 -> Out2/1

== system APF_CTL_VIS_Obs_2023a/Phase #3: Experiment/Change RED Behavior/Sub-Phase #4/GDC/Target Tracker/Constant Angular Rate ==
  state_black : Inport
  state_red : Inport  Port=2
  Looking Angle : MATLAB Function  TreatAsAtomicUnit=on
  theta_desired : Outport
  wires:
  Looking Angle/1(theta_desired) -> theta_desired/1
  state_black/1 -> Looking Angle/1(state_black)
  state_red/1 -> Looking Angle/2(state_red)

== system APF_CTL_VIS_Obs_2023a/Phase #3: Experiment/Change RED Behavior/Sub-Phase #4/GDC/Target Tracker/Hold Position ==
  Constant1 : Constant  Value=RED_ini(1)
  Constant2 : Constant  Value=RED_ini(2)
  Out1 : Outport
  Out2 : Outport  Port=2
  wires:
  Constant1/1 -> Out1/1
  Constant2/1 -> Out2/1

== system APF_CTL_VIS_Obs_2023a/Phase #3: Experiment/Change RED Behavior/Sub-Phase #4/RED+ARM/Simulated Position Controller/Custom Discrete PD (Elbow) ==
  ey : Inport
  Sum3 : Sum
  kd_elarm : Gain  Gain=Kd_elarm
  kp_elarm : Gain  Gain=Kp_elarm
  "x_dot -> x2" : Subsystem
  Fy : Outport  VectorParamsAs1DForOutWhenUnconnected=off
  wires:
  kd_elarm/1 -> Sum3/1
  Sum3/1 -> Fy/1
  kp_elarm/1 -> Sum3/2
  "x_dot -> x2"/1(dy(t)/dt) -> kd_elarm/1
  ey/1 -> "x_dot -> x2"/1(y(t)), kp_elarm/1

== system APF_CTL_VIS_Obs_2023a/Phase #3: Experiment/Change RED Behavior/Sub-Phase #4/RED+ARM/Simulated Position Controller/Custom Discrete PD (Shoulder) ==
  ex : Inport
  Sum3 : Sum
  kd_sharm : Gain  Gain=Kd_sharm
  kp_sharm : Gain  Gain=Kp_sharm
  "x_dot -> x2" : Subsystem
  Fx : Outport  VectorParamsAs1DForOutWhenUnconnected=off
  wires:
  kd_sharm/1 -> Sum3/1
  ex/1 -> "x_dot -> x2"/1(y(t)), kp_sharm/1
  kp_sharm/1 -> Sum3/2
  "x_dot -> x2"/1(dy(t)/dt) -> kd_sharm/1
  Sum3/1 -> Fx/1

== system APF_CTL_VIS_Obs_2023a/Phase #3: Experiment/Change RED Behavior/Sub-Phase #4/RED+ARM/Simulated Position Controller/Custom Discrete PD (Wrist) ==
  ey : Inport
  Sum3 : Sum
  kd_wrarm : Gain  Gain=Kd_wrarm
  kp_wrarm : Gain  Gain=Kp_wrarm
  "x_dot -> x2" : Subsystem
  Fy : Outport  VectorParamsAs1DForOutWhenUnconnected=off
  wires:
  kd_wrarm/1 -> Sum3/1
  Sum3/1 -> Fy/1
  kp_wrarm/1 -> Sum3/2
  "x_dot -> x2"/1(dy(t)/dt) -> kd_wrarm/1
  ey/1 -> "x_dot -> x2"/1(y(t)), kp_wrarm/1

== system APF_CTL_VIS_Obs_2023a/Phase #4: Return Home/Change RED Behavior/RED+ARM/Simulated Position Controller/Custom Discrete PD (Elbow)/x_dot -> x2 ==
  note: dy/dt ~= (y2-y1)/deltaT
  y(t) : Inport
  Delay1 : Delay  DelayLength=1  InitialConditionSource=Input port
      settings: InputPortMap=u0,p4
  Hold this value : Subsystem  TreatAsAtomicUnit=on
  Sum6 : Sum  Inputs=-+|
  divide by delta T : Gain  Gain=1/baseRate
  "if we went through a \"step\"" : If  IfExpression=u1 ~= 0  ShowElse=off
  dy(t)/dt : Outport  VectorParamsAs1DForOutWhenUnconnected=off
  wires:
  divide by delta T/1 -> dy(t)/dt/1
  Delay1/1 -> Sum6/1
  "if we went through a \"step\""/1 -> Hold this value/Action
  Hold this value/1(Out1) -> divide by delta T/1
  Sum6/1 -> "if we went through a \"step\""/1, Hold this value/1(In1)
  y(t)/1 -> Sum6/2, Delay1/2, Delay1/1

== system APF_CTL_VIS_Obs_2023a/Phase #4: Return Home/Change RED Behavior/RED+ARM/Simulated Position Controller/Custom Discrete PD (Shoulder)/x_dot -> x2 ==
  note: dy/dt ~= (y2-y1)/deltaT
  y(t) : Inport
  Delay1 : Delay  DelayLength=1  InitialConditionSource=Input port
      settings: InputPortMap=u0,p4
  Hold this value : Subsystem  TreatAsAtomicUnit=on
  Sum6 : Sum  Inputs=-+|
  divide by delta T : Gain  Gain=1/baseRate
  "if we went through a \"step\"" : If  IfExpression=u1 ~= 0  ShowElse=off
  dy(t)/dt : Outport  VectorParamsAs1DForOutWhenUnconnected=off
  wires:
  divide by delta T/1 -> dy(t)/dt/1
  Delay1/1 -> Sum6/1
  "if we went through a \"step\""/1 -> Hold this value/Action
  Hold this value/1(Out1) -> divide by delta T/1
  Sum6/1 -> "if we went through a \"step\""/1, Hold this value/1(In1)
  y(t)/1 -> Sum6/2, Delay1/2, Delay1/1

== system APF_CTL_VIS_Obs_2023a/Phase #4: Return Home/Change RED Behavior/RED+ARM/Simulated Position Controller/Custom Discrete PD (Wrist)/x_dot -> x2 ==
  note: dy/dt ~= (y2-y1)/deltaT
  y(t) : Inport
  Delay1 : Delay  DelayLength=1  InitialConditionSource=Input port
      settings: InputPortMap=u0,p4
  Hold this value : Subsystem  TreatAsAtomicUnit=on
  Sum6 : Sum  Inputs=-+|
  divide by delta T : Gain  Gain=1/baseRate
  "if we went through a \"step\"" : If  IfExpression=u1 ~= 0  ShowElse=off
  dy(t)/dt : Outport  VectorParamsAs1DForOutWhenUnconnected=off
  wires:
  divide by delta T/1 -> dy(t)/dt/1
  Delay1/1 -> Sum6/1
  "if we went through a \"step\""/1 -> Hold this value/Action
  Hold this value/1(Out1) -> divide by delta T/1
  Sum6/1 -> "if we went through a \"step\""/1, Hold this value/1(In1)
  y(t)/1 -> Sum6/2, Delay1/2, Delay1/1

== system APF_CTL_VIS_Obs_2023a/Phase #5: Hold Home/Change RED Behavior/RED+ARM/Simulated Position Controller/Custom Discrete PD (Elbow)/x_dot -> x2 ==
  note: dy/dt ~= (y2-y1)/deltaT
  y(t) : Inport
  Delay1 : Delay  DelayLength=1  InitialConditionSource=Input port
      settings: InputPortMap=u0,p4
  Hold this value : Subsystem  TreatAsAtomicUnit=on
  Sum6 : Sum  Inputs=-+|
  divide by delta T : Gain  Gain=1/baseRate
  "if we went through a \"step\"" : If  IfExpression=u1 ~= 0  ShowElse=off
  dy(t)/dt : Outport  VectorParamsAs1DForOutWhenUnconnected=off
  wires:
  divide by delta T/1 -> dy(t)/dt/1
  Delay1/1 -> Sum6/1
  "if we went through a \"step\""/1 -> Hold this value/Action
  Hold this value/1(Out1) -> divide by delta T/1
  Sum6/1 -> "if we went through a \"step\""/1, Hold this value/1(In1)
  y(t)/1 -> Sum6/2, Delay1/2, Delay1/1

== system APF_CTL_VIS_Obs_2023a/Phase #5: Hold Home/Change RED Behavior/RED+ARM/Simulated Position Controller/Custom Discrete PD (Shoulder)/x_dot -> x2 ==
  note: dy/dt ~= (y2-y1)/deltaT
  y(t) : Inport
  Delay1 : Delay  DelayLength=1  InitialConditionSource=Input port
      settings: InputPortMap=u0,p4
  Hold this value : Subsystem  TreatAsAtomicUnit=on
  Sum6 : Sum  Inputs=-+|
  divide by delta T : Gain  Gain=1/baseRate
  "if we went through a \"step\"" : If  IfExpression=u1 ~= 0  ShowElse=off
  dy(t)/dt : Outport  VectorParamsAs1DForOutWhenUnconnected=off
  wires:
  divide by delta T/1 -> dy(t)/dt/1
  Delay1/1 -> Sum6/1
  "if we went through a \"step\""/1 -> Hold this value/Action
  Hold this value/1(Out1) -> divide by delta T/1
  Sum6/1 -> "if we went through a \"step\""/1, Hold this value/1(In1)
  y(t)/1 -> Sum6/2, Delay1/2, Delay1/1

== system APF_CTL_VIS_Obs_2023a/Phase #5: Hold Home/Change RED Behavior/RED+ARM/Simulated Position Controller/Custom Discrete PD (Wrist)/x_dot -> x2 ==
  note: dy/dt ~= (y2-y1)/deltaT
  y(t) : Inport
  Delay1 : Delay  DelayLength=1  InitialConditionSource=Input port
      settings: InputPortMap=u0,p4
  Hold this value : Subsystem  TreatAsAtomicUnit=on
  Sum6 : Sum  Inputs=-+|
  divide by delta T : Gain  Gain=1/baseRate
  "if we went through a \"step\"" : If  IfExpression=u1 ~= 0  ShowElse=off
  dy(t)/dt : Outport  VectorParamsAs1DForOutWhenUnconnected=off
  wires:
  divide by delta T/1 -> dy(t)/dt/1
  Delay1/1 -> Sum6/1
  "if we went through a \"step\""/1 -> Hold this value/Action
  Hold this value/1(Out1) -> divide by delta T/1
  Sum6/1 -> "if we went through a \"step\""/1, Hold this value/1(In1)
  y(t)/1 -> Sum6/2, Delay1/2, Delay1/1

== system APF_CTL_VIS_Obs_2023a/Simulate Plant Dynamics/RED and ARM Dynamics/RED + ARM/RED + ARM Dynamics/x_dot -> x1/Hold this value ==
  In1 : Inport
  Action Port : ActionPort  ActionPortLabel=if(u1 ~= 0)
  Out1 : Outport  VectorParamsAs1DForOutWhenUnconnected=off
  wires:
  In1/1 -> Out1/1

== system APF_CTL_VIS_Obs_2023a/Simulate Plant Dynamics/RED and ARM Dynamics/RED + ARM/RED + ARM Dynamics/x_dot -> x2/Hold this value ==
  In1 : Inport
  Action Port : ActionPort  ActionPortLabel=if(u1 ~= 0)
  Out1 : Outport  VectorParamsAs1DForOutWhenUnconnected=off
  wires:
  In1/1 -> Out1/1

== system APF_CTL_VIS_Obs_2023a/Simulate Plant Dynamics/RED and ARM Dynamics/RED + ARM/RED + ARM Dynamics/x_dot -> x3/Hold this value ==
  In1 : Inport
  Action Port : ActionPort  ActionPortLabel=if(u1 ~= 0)
  Out1 : Outport  VectorParamsAs1DForOutWhenUnconnected=off
  wires:
  In1/1 -> Out1/1

== system APF_CTL_VIS_Obs_2023a/Simulate Plant Dynamics/RED and ARM Dynamics/RED Only/RED Dynamics/x_dot -> x1/Hold this value ==
  In1 : Inport
  Action Port : ActionPort  ActionPortLabel=if(u1 ~= 0)
  Out1 : Outport  VectorParamsAs1DForOutWhenUnconnected=off
  wires:
  In1/1 -> Out1/1

== system APF_CTL_VIS_Obs_2023a/Simulate Plant Dynamics/RED and ARM Dynamics/RED Only/RED Dynamics/x_dot -> x2/Hold this value ==
  In1 : Inport
  Action Port : ActionPort  ActionPortLabel=if(u1 ~= 0)
  Out1 : Outport  VectorParamsAs1DForOutWhenUnconnected=off
  wires:
  In1/1 -> Out1/1

== system APF_CTL_VIS_Obs_2023a/Simulate Plant Dynamics/RED and ARM Dynamics/RED Only/RED Dynamics/x_dot -> x3/Hold this value ==
  In1 : Inport
  Action Port : ActionPort  ActionPortLabel=if(u1 ~= 0)
  Out1 : Outport  VectorParamsAs1DForOutWhenUnconnected=off
  wires:
  In1/1 -> Out1/1

== system APF_CTL_VIS_Obs_2023a/Simulate Plant Dynamics/RED and ARM Dynamics/RED Only/RED Dynamics/x_dot -> x4/Hold this value ==
  In1 : Inport
  Action Port : ActionPort  ActionPortLabel=if(u1 ~= 0)
  Out1 : Outport  VectorParamsAs1DForOutWhenUnconnected=off
  wires:
  In1/1 -> Out1/1

== system APF_CTL_VIS_Obs_2023a/Simulate Plant Dynamics/RED and ARM Dynamics/RED Only/RED Dynamics/x_dot -> x5/Hold this value ==
  In1 : Inport
  Action Port : ActionPort  ActionPortLabel=if(u1 ~= 0)
  Out1 : Outport  VectorParamsAs1DForOutWhenUnconnected=off
  wires:
  In1/1 -> Out1/1

== system APF_CTL_VIS_Obs_2023a/Simulate Plant Dynamics/RED and ARM Dynamics/RED Only/RED Dynamics/x_dot -> x6/Hold this value ==
  In1 : Inport
  Action Port : ActionPort  ActionPortLabel=if(u1 ~= 0)
  Out1 : Outport  VectorParamsAs1DForOutWhenUnconnected=off
  wires:
  In1/1 -> Out1/1

== system APF_CTL_VIS_Obs_2023a/Phase #2: Initial Position/Change RED Behavior/RED+ARM/Simulated Position Controller/Custom Discrete PD (Elbow)/x_dot -> x2/Hold this value ==
  In1 : Inport
  Action Port : ActionPort  ActionPortLabel=if(u1 ~= 0)
  Out1 : Outport  VectorParamsAs1DForOutWhenUnconnected=off
  wires:
  In1/1 -> Out1/1

== system APF_CTL_VIS_Obs_2023a/Phase #2: Initial Position/Change RED Behavior/RED+ARM/Simulated Position Controller/Custom Discrete PD (Shoulder)/x_dot -> x2/Hold this value ==
  In1 : Inport
  Action Port : ActionPort  ActionPortLabel=if(u1 ~= 0)
  Out1 : Outport  VectorParamsAs1DForOutWhenUnconnected=off
  wires:
  In1/1 -> Out1/1

== system APF_CTL_VIS_Obs_2023a/Phase #2: Initial Position/Change RED Behavior/RED+ARM/Simulated Position Controller/Custom Discrete PD (Wrist)/x_dot -> x2/Hold this value ==
  In1 : Inport
  Action Port : ActionPort  ActionPortLabel=if(u1 ~= 0)
  Out1 : Outport  VectorParamsAs1DForOutWhenUnconnected=off
  wires:
  In1/1 -> Out1/1

== system APF_CTL_VIS_Obs_2023a/Phase #3: Experiment/Change RED Behavior/Sub-Phase #1/RED+ARM/Simulated Position Controller/Custom Discrete PD (Elbow)/x_dot -> x2 ==
  note: dy/dt ~= (y2-y1)/deltaT
  y(t) : Inport
  Delay1 : Delay  DelayLength=1  InitialConditionSource=Input port
      settings: InputPortMap=u0,p4
  Hold this value : Subsystem  TreatAsAtomicUnit=on
  Sum6 : Sum  Inputs=-+|
  divide by delta T : Gain  Gain=1/baseRate
  "if we went through a \"step\"" : If  IfExpression=u1 ~= 0  ShowElse=off
  dy(t)/dt : Outport  VectorParamsAs1DForOutWhenUnconnected=off
  wires:
  divide by delta T/1 -> dy(t)/dt/1
  Delay1/1 -> Sum6/1
  "if we went through a \"step\""/1 -> Hold this value/Action
  Hold this value/1(Out1) -> divide by delta T/1
  Sum6/1 -> "if we went through a \"step\""/1, Hold this value/1(In1)
  y(t)/1 -> Sum6/2, Delay1/2, Delay1/1

== system APF_CTL_VIS_Obs_2023a/Phase #3: Experiment/Change RED Behavior/Sub-Phase #1/RED+ARM/Simulated Position Controller/Custom Discrete PD (Shoulder)/x_dot -> x2 ==
  note: dy/dt ~= (y2-y1)/deltaT
  y(t) : Inport
  Delay1 : Delay  DelayLength=1  InitialConditionSource=Input port
      settings: InputPortMap=u0,p4
  Hold this value : Subsystem  TreatAsAtomicUnit=on
  Sum6 : Sum  Inputs=-+|
  divide by delta T : Gain  Gain=1/baseRate
  "if we went through a \"step\"" : If  IfExpression=u1 ~= 0  ShowElse=off
  dy(t)/dt : Outport  VectorParamsAs1DForOutWhenUnconnected=off
  wires:
  divide by delta T/1 -> dy(t)/dt/1
  Delay1/1 -> Sum6/1
  "if we went through a \"step\""/1 -> Hold this value/Action
  Hold this value/1(Out1) -> divide by delta T/1
  Sum6/1 -> "if we went through a \"step\""/1, Hold this value/1(In1)
  y(t)/1 -> Sum6/2, Delay1/2, Delay1/1

== system APF_CTL_VIS_Obs_2023a/Phase #3: Experiment/Change RED Behavior/Sub-Phase #1/RED+ARM/Simulated Position Controller/Custom Discrete PD (Wrist)/x_dot -> x2 ==
  note: dy/dt ~= (y2-y1)/deltaT
  y(t) : Inport
  Delay1 : Delay  DelayLength=1  InitialConditionSource=Input port
      settings: InputPortMap=u0,p4
  Hold this value : Subsystem  TreatAsAtomicUnit=on
  Sum6 : Sum  Inputs=-+|
  divide by delta T : Gain  Gain=1/baseRate
  "if we went through a \"step\"" : If  IfExpression=u1 ~= 0  ShowElse=off
  dy(t)/dt : Outport  VectorParamsAs1DForOutWhenUnconnected=off
  wires:
  divide by delta T/1 -> dy(t)/dt/1
  Delay1/1 -> Sum6/1
  "if we went through a \"step\""/1 -> Hold this value/Action
  Hold this value/1(Out1) -> divide by delta T/1
  Sum6/1 -> "if we went through a \"step\""/1, Hold this value/1(In1)
  y(t)/1 -> Sum6/2, Delay1/2, Delay1/1

== system APF_CTL_VIS_Obs_2023a/Phase #3: Experiment/Change RED Behavior/Sub-Phase #2 /RED+ARM/Simulated Position Controller/Custom Discrete PD (Elbow)/x_dot -> x2 ==
  note: dy/dt ~= (y2-y1)/deltaT
  y(t) : Inport
  Delay1 : Delay  DelayLength=1  InitialConditionSource=Input port
      settings: InputPortMap=u0,p4
  Hold this value : Subsystem  TreatAsAtomicUnit=on
  Sum6 : Sum  Inputs=-+|
  divide by delta T : Gain  Gain=1/baseRate
  "if we went through a \"step\"" : If  IfExpression=u1 ~= 0  ShowElse=off
  dy(t)/dt : Outport  VectorParamsAs1DForOutWhenUnconnected=off
  wires:
  divide by delta T/1 -> dy(t)/dt/1
  Delay1/1 -> Sum6/1
  "if we went through a \"step\""/1 -> Hold this value/Action
  Hold this value/1(Out1) -> divide by delta T/1
  Sum6/1 -> "if we went through a \"step\""/1, Hold this value/1(In1)
  y(t)/1 -> Sum6/2, Delay1/2, Delay1/1

== system APF_CTL_VIS_Obs_2023a/Phase #3: Experiment/Change RED Behavior/Sub-Phase #2 /RED+ARM/Simulated Position Controller/Custom Discrete PD (Shoulder)/x_dot -> x2 ==
  note: dy/dt ~= (y2-y1)/deltaT
  y(t) : Inport
  Delay1 : Delay  DelayLength=1  InitialConditionSource=Input port
      settings: InputPortMap=u0,p4
  Hold this value : Subsystem  TreatAsAtomicUnit=on
  Sum6 : Sum  Inputs=-+|
  divide by delta T : Gain  Gain=1/baseRate
  "if we went through a \"step\"" : If  IfExpression=u1 ~= 0  ShowElse=off
  dy(t)/dt : Outport  VectorParamsAs1DForOutWhenUnconnected=off
  wires:
  divide by delta T/1 -> dy(t)/dt/1
  Delay1/1 -> Sum6/1
  "if we went through a \"step\""/1 -> Hold this value/Action
  Hold this value/1(Out1) -> divide by delta T/1
  Sum6/1 -> "if we went through a \"step\""/1, Hold this value/1(In1)
  y(t)/1 -> Sum6/2, Delay1/2, Delay1/1
